simulink model "simu_MPC_MIMO"  (R2024b)
settings: Solver=VariableStepAuto  StartTime=0.0  StopTime=Tsim  RelTol=1e-3
values from neighbouring files (symbols this model uses):
  A = [A1, zeros(5) ... (first row only)    [bioreactor.m]    (also in mpc_mimo.m = [A1 zeros(size(A1)); zeros(size(A2)) A2])
  B = [B11(2:end), B12(2:end) ... (first row only)    [bioreactor.m]    (also in mpc_mimo.m = [B1 B2; B3 B4])
  D = 0    [bioreactor.m]    (also in mpc_mimo.m = [D1 zeros(size(D1)); zeros(size(D2)) D2])
  H = [H1, zeros(1, 5) ... (first row only)    [bioreactor.m]    (also in mpc_mimo.m = [H zeros(size(H)); zeros(size(H)) H])
  KE = K*E    [bioreactor.m]    (also in mpc_mimo.m)
  KF = K*F    [bioreactor.m]    (also in mpc_mimo.m)
  Kr = [sum(K(1, 1:2:2*N)), sum(K(1, 2:2:2*N)) ... (first row only)    [mpc_mimo.m]
  r1 = 0.35    [mpc_mimo.m]
  r1d = -0.1    [mpc_mimo.m]
  r2 = 0.06    [mpc_mimo.m]
  Tr1d = 50*Ts    (= 1.5)    [mpc_mimo.m]
undefined symbols (not defined in the file or in its folder): dist, Tdist
libraries: cstblocks x2
settings Model: Creator=sergio  LastModifiedBy=room2
settings RTWCC: GPUComputeCapability=3.5

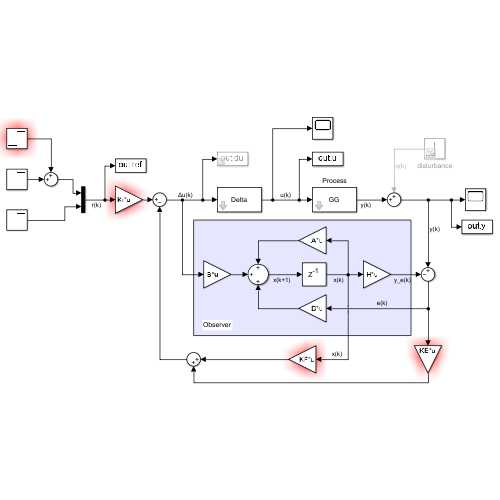
[thumbnail: Simulink's stored preview of the top-level diagram]
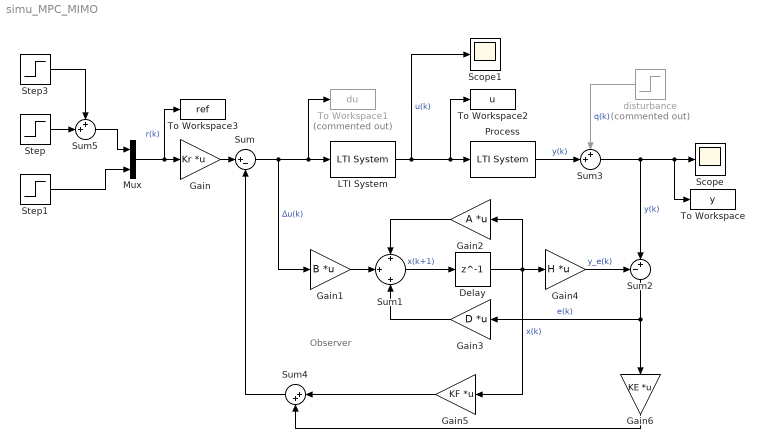
== system simu_MPC_MIMO ==
  note: Observer
  Delay : Delay  DelayLength=1
  Gain : Gain  Gain=Kr  Multiplication=Matrix(K*u)
  Gain1 : Gain  Gain=B  Multiplication=Matrix(K*u)
  Gain2 : Gain  Gain=A  Multiplication=Matrix(K*u)
  Gain3 : Gain  Gain=D  Multiplication=Matrix(K*u)
  Gain4 : Gain  Gain=H  Multiplication=Matrix(K*u)
  Gain5 : Gain  Gain=KF  Multiplication=Matrix(K*u)
  Gain6 : Gain  Gain=KE  Multiplication=Matrix(K*u)
  LTI System : cstblocks/LTI System  sys=Delta  IC=[]  PadeOrder=0
  Mux : Mux  Inputs=2
  Process : cstblocks/LTI System  sys=GG  IC=[]  PadeOrder=0
  Scope : Scope
  Scope1 : Scope
  Step : Step  Time=0  After=r1  SampleTime=0
  Step1 : Step  Time=0  After=r2  SampleTime=0
  Step3 : Step  Time=Tr1d  After=r1d  SampleTime=0
  Sum : Sum  Inputs=|+-
  Sum1 : Sum  Inputs=+|+|+
  Sum2 : Sum  Inputs=-+|
  Sum3 : Sum  Inputs=++|
  Sum4 : Sum  Inputs=|++
  Sum5 : Sum  Inputs=++|
  To Workspace : ToWorkspace  VariableName=y  SampleTime=-1
  To Workspace1 : ToWorkspace  Commented=on  VariableName=du  SampleTime=-1
  To Workspace2 : ToWorkspace  VariableName=u  SampleTime=-1
  To Workspace3 : ToWorkspace  VariableName=ref  SampleTime=-1
  disturbance : Step  Commented=on  Time=Tdist  After=dist  SampleTime=0
  wires:
  Sum/1 -> Gain1/1, To Workspace1/1, LTI System/1  "Δu(k)"
  LTI System/1 -> Scope1/1, To Workspace2/1, Process/1  "u(k)"
  Gain/1 -> Sum/1
  Gain1/1 -> Sum1/2
  Gain4/1 -> Sum2/1  "y_e(k)"
  Delay/1 -> Gain2/1, Gain5/1, Gain4/1  "x(k)"
  Sum1/1 -> Delay/1  "x(k+1)"
  Sum2/1 -> Gain3/1, Gain6/1  "e(k)"
  Gain2/1 -> Sum1/1
  Gain3/1 -> Sum1/3
  Process/1 -> Sum3/2  "y(k)"
  Sum3/1 -> Sum2/2, To Workspace/1, Scope/1  "y(k)"
  disturbance/1 -> Sum3/1  "q(k)"
  Mux/1 -> To Workspace3/1, Gain/1  "r(k)"
  Step1/1 -> Mux/2
  Sum4/1 -> Sum/2
  Gain5/1 -> Sum4/1
  Gain6/1 -> Sum4/2
  Step/1 -> Sum5/2
  Sum5/1 -> Mux/1
  Step3/1 -> Sum5/1
